simulink model "fangbo_pll_eso_J_identification"  (R2018b)
settings: Solver=FixedStepAuto  StartTime=0.0  StopTime=0.2  FixedStep=1e-7  RelTol=1e-3
InitFcn:
  | Vin1=30;%注入高频信号幅值
  | fin1=5000;%注入高频信号频率
  | fpwm=10000;%电流环控制频率
  | Tpwm=1/fpwm;
  | Tspd=Tpwm*10;%速度环控制周期（未用）
  | Td=2e-6;%逆变器死区时间（未加入）
  | Udc=90;
  | Pn=4;%极对数
  | R=0.281;
  | Ld=2.523e-3;Lq=5e-3;
  | faif=0.13455;
  | J=0.0012145+ 0.00126+0.0002601;%两个电机加联轴器
  | B=0.0006;
  | TL=10;%额定负载
  | nref=2200;%给定转速
  | %%%%%%luenberger观测器参数%%%%%%%
  | p=2*pi*10;%2;%极点位置，可调
  | eta=1;%1e-2;
  | alpha1=3*p;
  | alpha2=3*p^2;
  | alpha3=p^3;
  | %%%%%%锁相环参数%%%%%%%%%%%%%%%%%
  | Kppll= 300;   %2*p
  | Kipll= 1000;  %p^2
  | %%%%%%%%%双闭环3对PI参数%%%%%%%%%
  | BWc=300*2*pi;%电流环带宽
  | h=6;%速度环中频宽
  | K1=9.55*1.5*Pn*faif/J;
  | wcon=200*2*pi;%转速环反馈滤波和给定滤波器截止频率
  | Tsn=1/BWc+1/wcon;
  | Kpd=BWc*Ld;
  | Kid=R/Ld;
  | Kpq=BWc*Lq;
  | Kiq=R/Lq;
  | Kps=(h+1)/(2*h*Tsn*K1);
  | Kis=1/(h*Tsn);
  | %BWs=15*2*pi;
  | %Kps=BWs/K1;
  | %Kis=Kps*BWs/5;
  | %%%%%%%%%%%扰动观测器PID参数%%%%%%%%%%%%%
  | pd=2*pi*50;
  | kd_d=3*pd;
  | kp_d=3*pd^2;
  | ki_d=pd^3;
undefined symbols (not defined in the file): DiscIntNeverNeededParam, fin
libraries: simulink x16, dsparch4 x7, powerlib x5, dspsrcs4 x2, powerlib_meascontrol x2
(part 2 of 2)

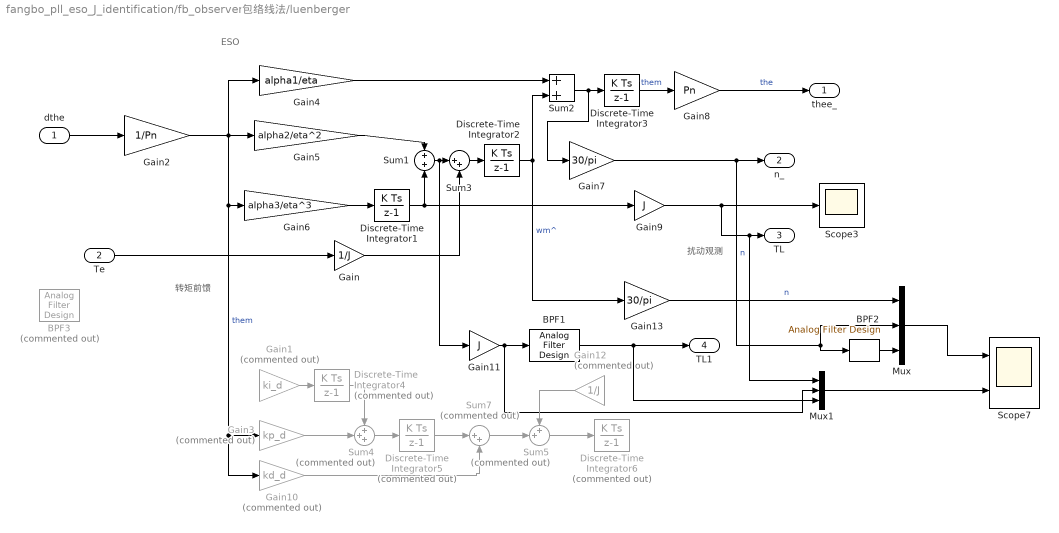
== system fangbo_pll_eso_J_identification/fb_observer包络线法/luenberger ==
  note: 转矩前馈
  note: ESO
  note: 扰动观测
  dthe : Inport
  Te : Inport  Port=2
  BPF1 : dsparch4/Analog Filter Design  method=Butterworth  filttype=Lowpass  N=2  Wlo=100*2*pi  Whi=(fin+200)*2*pi  Rp=2  Rs=40
  BPF2 : dsparch4/Analog Filter Design  method=Butterworth  filttype=Lowpass  N=1  Wlo=wcon  Whi=(fin+200)*2*pi  Rp=2  Rs=40
  BPF3 : dsparch4/Analog Filter Design  Commented=on  method=Butterworth  filttype=Lowpass  N=1  Wlo=100*2*pi  Whi=(fin+200)*2*pi  Rp=2  Rs=40
  Discrete-Time Integrator1 : DiscreteIntegrator  SampleTime=Tpwm  ICPrevOutput=DiscIntNeverNeededParam  ICPrevScaledInput=DiscIntNeverNeededParam
  Discrete-Time Integrator2 : DiscreteIntegrator  SampleTime=Tpwm  ICPrevOutput=DiscIntNeverNeededParam  ICPrevScaledInput=DiscIntNeverNeededParam
  Discrete-Time Integrator3 : DiscreteIntegrator  SampleTime=Tpwm  ICPrevOutput=DiscIntNeverNeededParam  ICPrevScaledInput=DiscIntNeverNeededParam
  Discrete-Time Integrator4 : DiscreteIntegrator  Commented=on  SampleTime=Tpwm  ICPrevOutput=DiscIntNeverNeededParam  ICPrevScaledInput=DiscIntNeverNeededParam
  Discrete-Time Integrator5 : DiscreteIntegrator  Commented=on  SampleTime=Tpwm  ICPrevOutput=DiscIntNeverNeededParam  ICPrevScaledInput=DiscIntNeverNeededParam
  Discrete-Time Integrator6 : DiscreteIntegrator  Commented=on  SampleTime=Tpwm  ICPrevOutput=DiscIntNeverNeededParam  ICPrevScaledInput=DiscIntNeverNeededParam
  Gain : Gain  Gain=1/J
  Gain1 : Gain  Commented=on  Gain=ki_d
  Gain10 : Gain  Commented=on  Gain=kd_d
  Gain11 : Gain  Gain=J
  Gain12 : Gain  Commented=on  Gain=1/J
  Gain13 : Gain  Gain=30/pi
  Gain2 : Gain  Gain=1/Pn
  Gain3 : Gain  Commented=on  Gain=kp_d
  Gain4 : Gain  Gain=alpha1/eta
  Gain5 : Gain  Gain=alpha2/eta^2
  Gain6 : Gain  Gain=alpha3/eta^3
  Gain7 : Gain  Gain=30/pi
  Gain8 : Gain  Gain=Pn
  Gain9 : Gain  Gain=J
  Mux : Mux  Inputs=3
  Mux1 : Mux  Inputs=3
  Scope3 : Scope
  Scope7 : Scope  NumInputPorts=2
  Sum1 : Sum  Inputs=+|+
  Sum2 : Sum
  Sum3 : Sum  Inputs=|++
  Sum4 : Sum  Commented=on  Inputs=+++
  Sum5 : Sum  Commented=on  Inputs=++|
  Sum7 : Sum  Commented=on  Inputs=|++
  thee_ : Outport
  n_ : Outport  Port=2
  TL : Outport  Port=3
  TL1 : Outport  Port=4
  wires:
  Gain7/1 -> BPF2/1, Mux/2, n_/1  "n"
  Gain9/1 -> Mux1/1, TL/1, Scope3/1
  Gain2/1 -> Gain4/1, Gain5/1, Gain10/1, Gain3/1, Gain6/1  "them"
  Gain5/1 -> Sum1/1
  Te/1 -> Gain/1
  Gain6/1 -> Discrete-Time Integrator1/1
  Discrete-Time Integrator1/1 -> Sum1/2, Gain9/1
  Sum2/1 -> Gain7/1, Discrete-Time Integrator3/1
  Sum1/1 -> Gain11/1, Sum3/1
  Gain/1 -> Sum3/2
  Gain4/1 -> Sum2/1
  Discrete-Time Integrator2/1 -> Gain13/1, Sum2/2  "wm^"
  Gain8/1 -> thee_/1  "the"
  Discrete-Time Integrator3/1 -> Gain8/1  "them"
  dthe/1 -> Gain2/1
  Gain1/1 -> Discrete-Time Integrator4/1
  Gain3/1 -> Sum4/2
  Gain10/1 -> Sum7/2
  Sum7/1 -> Sum5/2
  Gain11/1 -> Mux1/2, BPF1/1
  Gain12/1 -> Sum5/1
  Sum5/1 -> Discrete-Time Integrator6/1
  Mux/1 -> Scope7/1
  Mux1/1 -> Scope7/2
  Discrete-Time Integrator4/1 -> Sum4/1
  Discrete-Time Integrator5/1 -> Sum7/1
  Sum4/1 -> Discrete-Time Integrator5/1
  Sum3/1 -> Discrete-Time Integrator2/1
  BPF1/1 -> Mux1/3, TL1/1
  Gain13/1 -> Mux/1  "n"
  BPF2/1 -> Mux/3

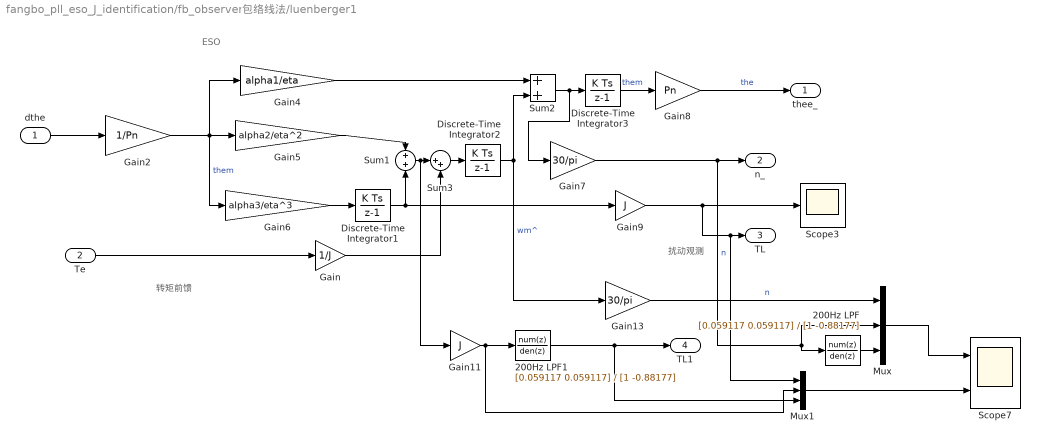
== system fangbo_pll_eso_J_identification/fb_observer包络线法/luenberger1 ==
  note: 扰动观测
  note: ESO
  note: 转矩前馈
  dthe : Inport
  Te : Inport  Port=2
  200Hz LPF : DiscreteTransferFcn  Numerator=[0.059117 0.059117]  Denominator=[1 -0.88177]  SampleTime=Tpwm
  200Hz LPF1 : DiscreteTransferFcn  Numerator=[0.059117 0.059117]  Denominator=[1 -0.88177]  SampleTime=Tpwm
  Discrete-Time Integrator1 : DiscreteIntegrator  SampleTime=Tpwm  ICPrevOutput=DiscIntNeverNeededParam  ICPrevScaledInput=DiscIntNeverNeededParam
  Discrete-Time Integrator2 : DiscreteIntegrator  SampleTime=Tpwm  ICPrevOutput=DiscIntNeverNeededParam  ICPrevScaledInput=DiscIntNeverNeededParam
  Discrete-Time Integrator3 : DiscreteIntegrator  SampleTime=Tpwm  ICPrevOutput=DiscIntNeverNeededParam  ICPrevScaledInput=DiscIntNeverNeededParam
  Gain : Gain  Gain=1/J
  Gain11 : Gain  Gain=J
  Gain13 : Gain  Gain=30/pi
  Gain2 : Gain  Gain=1/Pn
  Gain4 : Gain  Gain=alpha1/eta
  Gain5 : Gain  Gain=alpha2/eta^2
  Gain6 : Gain  Gain=alpha3/eta^3
  Gain7 : Gain  Gain=30/pi
  Gain8 : Gain  Gain=Pn
  Gain9 : Gain  Gain=J
  Mux : Mux  Inputs=3
  Mux1 : Mux  Inputs=3
  Scope3 : Scope
  Scope7 : Scope  NumInputPorts=2
  Sum1 : Sum  Inputs=+|+
  Sum2 : Sum
  Sum3 : Sum  Inputs=|++
  thee_ : Outport
  n_ : Outport  Port=2
  TL : Outport  Port=3
  TL1 : Outport  Port=4
  wires:
  200Hz LPF/1 -> Mux/3
  Gain13/1 -> Mux/1  "n"
  200Hz LPF1/1 -> TL1/1, Mux1/3
  Sum3/1 -> Discrete-Time Integrator2/1
  Mux1/1 -> Scope7/2
  Mux/1 -> Scope7/1
  Gain11/1 -> 200Hz LPF1/1, Mux1/2
  dthe/1 -> Gain2/1
  Discrete-Time Integrator3/1 -> Gain8/1  "them"
  Gain8/1 -> thee_/1  "the"
  Discrete-Time Integrator2/1 -> Sum2/2, Gain13/1  "wm^"
  Gain4/1 -> Sum2/1
  Gain/1 -> Sum3/2
  Sum1/1 -> Sum3/1, Gain11/1
  Sum2/1 -> Discrete-Time Integrator3/1, Gain7/1
  Discrete-Time Integrator1/1 -> Gain9/1, Sum1/2
  Gain6/1 -> Discrete-Time Integrator1/1
  Te/1 -> Gain/1
  Gain5/1 -> Sum1/1
  Gain2/1 -> Gain6/1, Gain5/1, Gain4/1  "them"
  Gain9/1 -> Scope3/1, TL/1, Mux1/1
  Gain7/1 -> n_/1, 200Hz LPF/1, Mux/2  "n"

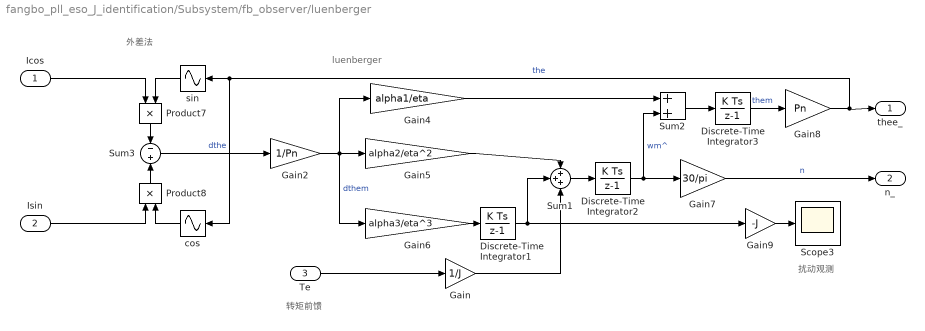
== system fangbo_pll_eso_J_identification/Subsystem/fb_observer/luenberger ==
  note: 转矩前馈
  note: luenberger
  note: 外差法
  note: 扰动观测
  Icos : Inport
  Isin : Inport  Port=2
  Te : Inport  Port=3
  Discrete-Time Integrator1 : DiscreteIntegrator  SampleTime=Tpwm  ICPrevOutput=DiscIntNeverNeededParam  ICPrevScaledInput=DiscIntNeverNeededParam
  Discrete-Time Integrator2 : DiscreteIntegrator  SampleTime=Tpwm  ICPrevOutput=DiscIntNeverNeededParam  ICPrevScaledInput=DiscIntNeverNeededParam
  Discrete-Time Integrator3 : DiscreteIntegrator  SampleTime=Tpwm  ICPrevOutput=DiscIntNeverNeededParam  ICPrevScaledInput=DiscIntNeverNeededParam
  Gain : Gain  Gain=1/J
  Gain2 : Gain  Gain=1/Pn
  Gain4 : Gain  Gain=alpha1/eta
  Gain5 : Gain  Gain=alpha2/eta^2
  Gain6 : Gain  Gain=alpha3/eta^3
  Gain7 : Gain  Gain=30/pi
  Gain8 : Gain  Gain=Pn
  Gain9 : Gain  Gain=-J
  Product7 : Product
  Product8 : Product
  Scope3 : Scope
  Sum1 : Sum  Inputs=+++
  Sum2 : Sum
  Sum3 : Sum  Inputs=-|+
  cos : Sin  TimeSource=Use external signal  Phase=pi/2  SampleTime=0
  sin : Sin  TimeSource=Use external signal  SampleTime=0
  thee_ : Outport
  n_ : Outport  Port=2
  wires:
  Gain7/1 -> n_/1  "n"
  Gain9/1 -> Scope3/1
  Icos/1 -> Product7/1
  Isin/1 -> Product8/1
  Gain2/1 -> Gain4/1, Gain5/1, Gain6/1  "dthem"
  Gain5/1 -> Sum1/1
  Te/1 -> Gain/1
  Gain6/1 -> Discrete-Time Integrator1/1
  Discrete-Time Integrator1/1 -> Sum1/2, Gain9/1
  Sum2/1 -> Discrete-Time Integrator3/1
  Sum1/1 -> Discrete-Time Integrator2/1
  Gain/1 -> Sum1/3
  Gain4/1 -> Sum2/1
  Discrete-Time Integrator2/1 -> Sum2/2, Gain7/1  "wm^"
  Sum3/1 -> Gain2/1  "dthe"
  Gain8/1 -> thee_/1, cos/1, sin/1  "the"
  Product7/1 -> Sum3/1
  Discrete-Time Integrator3/1 -> Gain8/1  "them"
  Product8/1 -> Sum3/2
  cos/1 -> Product8/2
  sin/1 -> Product7/2

== matlab function fangbo_pll_eso_J_identification/MATLAB Function1 ==
  settings: updateMethod=DISCRETE
  data: u input size=[1 4]; y output size=[1 2]
function y = fcn(u)
%基于ESO的自抗扰控制器 参考刘慧贤博士学位论文 《永磁同步电机交流伺服系统的非线性控制算法研究》
% 输入： u(1)转速 n(k) n/min; u(2)电流iq(k-1); u(3)为ADRC_w(k-1); u(4)为ADRC_iq(k-1);
% 输出： y(1) 估计的转速 ；y(2)估计的扰动
T = 0.0001;
p = 2*pi*30;
b0 = 1.5*4*0.13455*400; % 电磁转矩系数 
nk = u(1)*pi/30; %转速转化为机械角速度 rad/s
wk_1 = u(3)*pi/30; %转速转化为机械角速度 rad/s
u(4) = u(4)*b0;
%persistent wk
%if isempty(wk)
%    wk = 0;end
%persistent iqk
%if isempty(iqk)
%    iqk = 0;end
wk = wk_1 + T*u(4) - T*2*p*(wk_1 - nk) + T*b0*u(2);
iqk = u(4) - T*p*p*(wk_1 - nk);
y = [wk*30/pi iqk/b0];

== matlab function fangbo_pll_eso_J_identification/MATLAB Function ==
  settings: updateMethod=DISCRETE
  data: u input size=[1 2]; y output size=[1 2]
function y = fcn(u)
%基于ESO的自抗扰控制器 参考刘慧贤博士学位论文 《永磁同步电机交流伺服系统的非线性控制算法研究》
% 输入： u(1)转速 w(k) rad/s ; u(2) iq*(k-1)
% 输出： y(1) 估计的转速 ；y(2)估计的扰动
u(1) = u(1)*pi/30; %转速转化为机械角速度
persistent z1_0
if isempty(z1_0)
    z1_0 = 0;end
persistent z1_1
if isempty(z1_1)
    z1_1 = 0;end
persistent z2_0
if isempty(z2_0)
    z2_0 = 0;end
persistent z2_1
if isempty(z2_1)
    z2_1 = 0;end
persistent iq_1
if isempty(iq_1)
    iq_1 = 0;end
T = 0.0001;
p = 2*pi*40;
b0 = 1.5*4*0.13455*400; % 电磁转矩系数 
z1_0 = z1_1 + T*z2_1 - T*2*p*(z1_1 - u(1)) + T*b0*iq_1;
z2_0 = z2_1 - T*p*p*(z1_1 - u(1));
z1_1 = z1_0;
z2_1 = z2_0;
iq_1 = u(2); %保存上一时刻的q轴电流参考值
y = [z1_0*30/pi z2_0/b0];

== matlab function fangbo_pll_eso_J_identification/MATLAB Function2 ==
  data: x1 input size=[2 1]; y1 output size=[2 1]; x2 input size=[2 2]; x3 input; x4 input; y2 output size=[2 1]; y3 output size=[2 2]; x5 input
function [y1,y2,y3]  = fcn(x1,x2,x3,x4,x5)
%转动惯量和转矩辨识
%输入 x3 iq*KT = 1.5*p*Ψf*iq; x4 转速微分 dw = [w(k) - w(k+1)]/T ; x5 阶跃信号 初始化用
%输入 x1  theta(k-1) 2×1;   x2  P(k-1) 2×2;
%输出 y1  theta(k) 2×1;   y2   K(k) 2×1;    y3  P(k) 2×2;
n = 20; %初始化的数组长度
persistent array
if isempty(array)
    array = ones(2,n);end
persistent array_Te
if isempty(array_Te)
    array_Te = zeros(n,1);end
if(x5<=0)
    thetaK_1 = x1;
    PK_1 = x2;
    for i=1:(n-1)
        array(1,i) = array(1,i+1);
        array_Te(i,1) = array_Te(i+1,1);
    end 
    array(1,n) = x4;
    array_Te(n,1) = x3; 
else
    thetaK_1 = inv(array*array')*array*array_Te;  %计算初值
    PK_1 = inv(array*array');
end
lambda = 0.9; %一般取[0.95,0.99]
KK = PK_1*[x4;1]/(lambda+[x4 1]*PK_1*[x4;1]);
thetaK = thetaK_1 + KK*(x3-[x4 1]*thetaK_1);
PK = ([1 0;0 1]-KK*[x4 1])*PK_1/lambda;
y1 = thetaK;
y2 = KK;
y3 = PK;
end
